simulink model "prescan_repl_modifyInputs"  (R2019a)
settings: Solver=VariableStepAuto  StartTime=0.0  StopTime=100  RelTol=1e-3
libraries: ProSivic_Sensors x2, realtime_pacer_lib x1
settings Model: Creator=Markus Borg  LastModifiedBy=Markus Borg

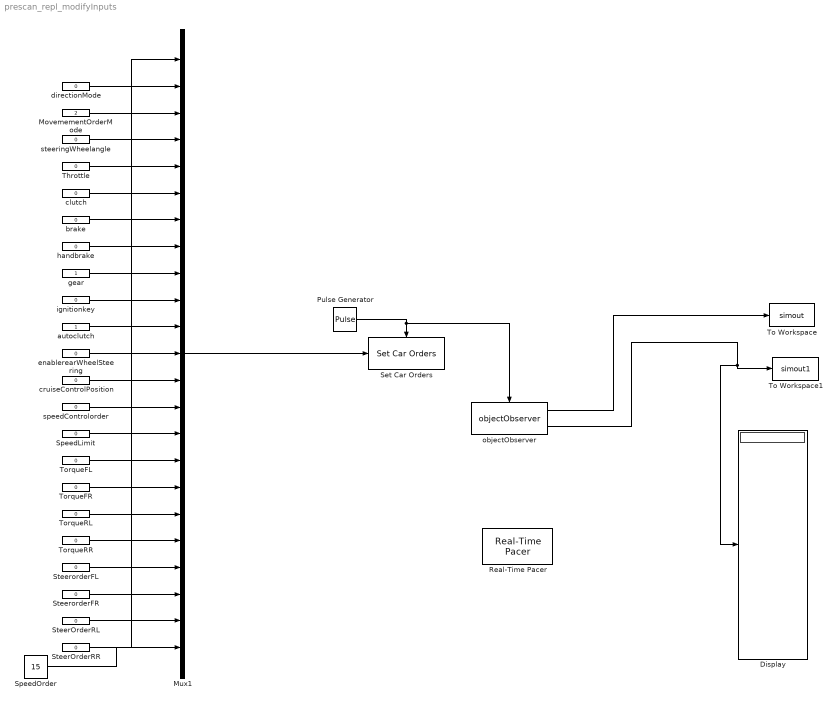
== system prescan_repl_modifyInputs ==
  Display : Display
  MovemementOrderMode : Constant  Value=2
  Mux1 : Mux  Inputs=23
  Pulse Generator : DiscretePulseGenerator  PulseType=Time based  Period=0.5  PulseWidth=50
  Real-Time Pacer : realtime_pacer_lib/Real-Time Pacer  simTimePerRealTime=inf
  Set Car Orders : ProSivic_Sensors/Set Car Orders  topic=Vehicle/car
  SpeedLimit : Constant  Value=0
  SpeedOrder : Constant  Value=15
  SteerOrderRL : Constant  Value=0
  SteerOrderRR : Constant  Value=0
  SteerorderFL : Constant  Value=0
  SteerorderFR : Constant  Value=0
  Throttle : Constant  Value=0
  To Workspace : ToWorkspace  VariableName=simout  SaveFormat=Timeseries  SampleTime=-1
  To Workspace1 : ToWorkspace  VariableName=simout1  SaveFormat=Timeseries  SampleTime=-1
  TorqueFL : Constant  Value=0
  TorqueFR : Constant  Value=0
  TorqueRL : Constant  Value=0
  TorqueRR : Constant  Value=0
  autoclutch : Constant
  brake : Constant  Value=0
  clutch : Constant  Value=0
  cruiseControlPosition : Constant  Value=0
  directionMode : Constant  Value=0
  enablerearWheelSteering : Constant  Value=0
  gear : Constant
  handbrake : Constant  Value=0
  ignitionkey : Constant  Value=0
  objectObserver : ProSivic_Sensors/objectObserver  topic=test
  speedControlorder : Constant  Value=0
  steeringWheelangle : Constant  Value=0
  wires:
  objectObserver/1 -> To Workspace/1
  Pulse Generator/1 -> objectObserver/Trigger, Set Car Orders/Trigger
  Mux1/1 -> Set Car Orders/1
  ignitionkey/1 -> Mux1/9
  SteerorderFR/1 -> Mux1/20
  SteerorderFL/1 -> Mux1/19
  TorqueFL/1 -> Mux1/15
  TorqueRL/1 -> Mux1/17
  speedControlorder/1 -> Mux1/13
  TorqueRR/1 -> Mux1/18
  Throttle/1 -> Mux1/4
  cruiseControlPosition/1 -> Mux1/12
  autoclutch/1 -> Mux1/10
  SteerOrderRL/1 -> Mux1/21
  enablerearWheelSteering/1 -> Mux1/11
  SpeedLimit/1 -> Mux1/14
  SpeedOrder/1 -> Mux1/23
  brake/1 -> Mux1/6
  MovemementOrderMode/1 -> Mux1/2
  gear/1 -> Mux1/8
  directionMode/1 -> Mux1/1
  steeringWheelangle/1 -> Mux1/3
  clutch/1 -> Mux1/5
  handbrake/1 -> Mux1/7
  TorqueFR/1 -> Mux1/16
  SteerOrderRR/1 -> Mux1/22
  objectObserver/2 -> Display/1, To Workspace1/1
